simulink subsystem "Multiple_ECG_Signal_QRS_Detector_With_Tunable_Bandpass"  (R2021a)
settings: Solver=VariableStepAuto  StartTime=0.0  StopTime=10.0  RelTol=1e-3
libraries: QRS_Detector_Library x7
settings Model: Creator=wallyproenza  LastModifiedBy=wallyproenza

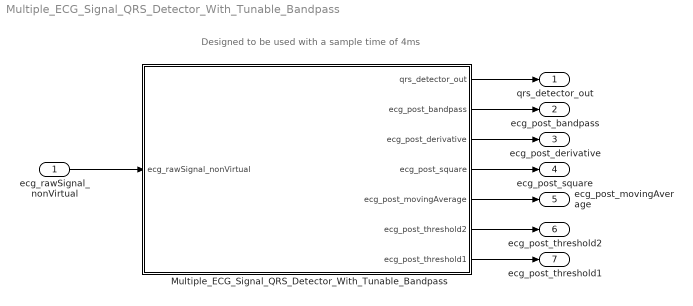
== system Multiple_ECG_Signal_QRS_Detector_With_Tunable_Bandpass ==
  note: Designed to be used with a sample time of 4ms
  ecg_rawSignal_nonVirtual : Inport
  Multiple_ECG_Signal_QRS_Detector_With_Tunable_Bandpass : Subsystem  TreatAsAtomicUnit=on
  qrs_detector_out : Outport
  ecg_post_bandpass : Outport  Port=2
  ecg_post_derivative : Outport  Port=3
  ecg_post_square : Outport  Port=4
  ecg_post_movingAverage : Outport  Port=5
  ecg_post_threshold2 : Outport  Port=6
  ecg_post_threshold1 : Outport  Port=7
  wires:
  ecg_rawSignal_nonVirtual/1 -> Multiple_ECG_Signal_QRS_Detector_With_Tunable_Bandpass/1(ecg_rawSignal_nonVirtual)
  Multiple_ECG_Signal_QRS_Detector_With_Tunable_Bandpass/3(ecg_post_derivative) -> ecg_post_derivative/1
  Multiple_ECG_Signal_QRS_Detector_With_Tunable_Bandpass/6(ecg_post_threshold2) -> ecg_post_threshold2/1
  Multiple_ECG_Signal_QRS_Detector_With_Tunable_Bandpass/2(ecg_post_bandpass) -> ecg_post_bandpass/1
  Multiple_ECG_Signal_QRS_Detector_With_Tunable_Bandpass/7(ecg_post_threshold1) -> ecg_post_threshold1/1
  Multiple_ECG_Signal_QRS_Detector_With_Tunable_Bandpass/5(ecg_post_movingAverage) -> ecg_post_movingAverage/1
  Multiple_ECG_Signal_QRS_Detector_With_Tunable_Bandpass/4(ecg_post_square) -> ecg_post_square/1
  Multiple_ECG_Signal_QRS_Detector_With_Tunable_Bandpass/1(qrs_detector_out) -> qrs_detector_out/1

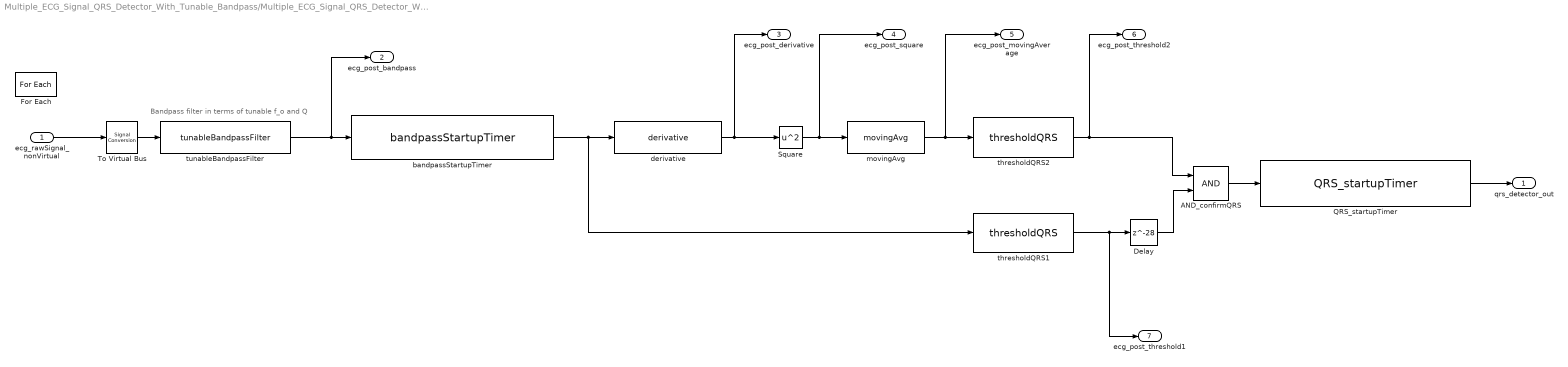
== system Multiple_ECG_Signal_QRS_Detector_With_Tunable_Bandpass/Multiple_ECG_Signal_QRS_Detector_With_Tunable_Bandpass ==
  note: Bandpass filter in terms of tunable f_o and Q
  ecg_rawSignal_nonVirtual : Inport  Partition=on  PartitionDimension=1  PartitionWidth=1  PartitionOffset=0
  AND_confirmQRS : Logic  IconShape=distinctive  AllPortsSameDT=off  OutDataTypeStr=boolean
  Delay : Delay  DelayLength=28  InitialCondition=0
  For Each : ForEach  DisableCoverage=on
  QRS_startupTimer : QRS_Detector_Library/QRS_startupTimer  SystemSampleTime=-1  VariantActivationTime=update diagram  Latency=0  AutoFrameSizeCalculation=off
  Square : Math  Operator=square  SaturateOnIntegerOverflow=on
  To Virtual Bus : SignalConversion  ConversionOutput=Virtual bus  OverrideOpt=off
  bandpassStartupTimer : QRS_Detector_Library/bandpassStartupTimer  SystemSampleTime=-1  VariantActivationTime=update diagram  Latency=0  AutoFrameSizeCalculation=off
  derivative : QRS_Detector_Library/derivative  SystemSampleTime=-1  VariantActivationTime=update diagram  Latency=0  AutoFrameSizeCalculation=off
  movingAvg : QRS_Detector_Library/movingAvg  SystemSampleTime=-1  VariantActivationTime=update diagram  Latency=0  AutoFrameSizeCalculation=off
  thresholdQRS1 : QRS_Detector_Library/thresholdQRS  SystemSampleTime=-1  VariantActivationTime=update diagram  Latency=0  AutoFrameSizeCalculation=off
  thresholdQRS2 : QRS_Detector_Library/thresholdQRS  SystemSampleTime=-1  VariantActivationTime=update diagram  Latency=0  AutoFrameSizeCalculation=off
  tunableBandpassFilter : QRS_Detector_Library/tunableBandpassFilter  SystemSampleTime=-1  VariantActivationTime=update diagram  Latency=0  AutoFrameSizeCalculation=off
  qrs_detector_out : Outport  ConcatenationDimension=1
  ecg_post_bandpass : Outport  Port=2  ConcatenationDimension=1
  ecg_post_derivative : Outport  Port=3  ConcatenationDimension=1
  ecg_post_square : Outport  Port=4  ConcatenationDimension=1
  ecg_post_movingAverage : Outport  Port=5  ConcatenationDimension=1
  ecg_post_threshold2 : Outport  Port=6  ConcatenationDimension=1
  ecg_post_threshold1 : Outport  Port=7  ConcatenationDimension=1
  wires:
  QRS_startupTimer/1 -> qrs_detector_out/1
  AND_confirmQRS/1 -> QRS_startupTimer/1
  bandpassStartupTimer/1 -> derivative/1, thresholdQRS1/1
  tunableBandpassFilter/1 -> ecg_post_bandpass/1, bandpassStartupTimer/1
  To Virtual Bus/1 -> tunableBandpassFilter/1
  Square/1 -> ecg_post_square/1, movingAvg/1
  thresholdQRS1/1 -> ecg_post_threshold1/1, Delay/1
  Delay/1 -> AND_confirmQRS/2
  thresholdQRS2/1 -> ecg_post_threshold2/1, AND_confirmQRS/1
  derivative/1 -> Square/1, ecg_post_derivative/1
  movingAvg/1 -> ecg_post_movingAverage/1, thresholdQRS2/1
  ecg_rawSignal_nonVirtual/1 -> To Virtual Bus/1
